simulink model "wireless_networked_control_HIL"  (Simulink 10.2)
settings: Solver=ode4  StartTime=0.0  StopTime=TfR  FixedStep=delta_t  RelTol=1e-3  EnableMultiTasking=on
values from neighbouring files (symbols this model uses):
  A1 = 0.01    [CoupledTanks_state_main.m]    (also in CoupledTanks_state_main_noise.m)
  A2 = 0.006    [CoupledTanks_state_main.m]    (also in CoupledTanks_state_main_noise.m)
  A3 = 0.12    [CoupledTanks_state_main.m]    (also in CoupledTanks_state_main_noise.m)
  A4 = 0.007    [CoupledTanks_state_main.m]    (also in CoupledTanks_state_main_noise.m)
  alpha1 = 10    [CoupledTanks_state_main.m]    (also in CoupledTanks_state_main_noise.m)
  AR = 1    [Controllersfun.m]    (also in Controllersfun2.m; CoupledTanks_state_main.m; CoupledTanks_state_main_noise.m)
  AR1 = 1    [CoupledTanks_state_main.m]    (also in CoupledTanks_state_main_noise.m)
  Atrace = [link5f(yh*trace_count+1:(yh+1)*trace_count+200),     link2f(yh*trace_count+1:(yh+1)*trace_count+200),     link3f(yh*trace_count+1:(yh+1)*trace_count+200),     link8f(yh*trace_count+1:(yh+1)*trace_count+200)]    [CoupledTanks_state_main.m]    (also in CoupledTanks_state_main_noise.m = Atrace_first_half; Mediasfun.m = Atrace_second_half)
  delta_t = 1/system_rate    (= 0.00104166666667)    [CoupledTanks_state_main.m]    (also in CoupledTanks_state_main_noise.m)
  delta_tc = abs(randn(N,1))    [ADPS_fig2_execution_timeanalyse.m]    (also in CoupledTanks_state_main.m = 0.0416666666667; CoupledTanks_state_main_noise.m = 0.0416666666667)
  delta_tc2 = 1/sensing_rate2    (= 0.0416666666667)    [CoupledTanks_state_main.m]    (also in CoupledTanks_state_main_noise.m)
  delta_tr = 8/960    (= 0.00833333333333)    [CoupledTanks_state_main.m]    (also in CoupledTanks_state_main_noise.m)
  g = 9.8    [Controllersfun.m]    (also in Controllersfun2.m; CoupledTanks_state_main.m; CoupledTanks_state_main_noise.m; EKFsfun.m)
  L1ini = 6    [CoupledTanks_state_main.m]    (also in CoupledTanks_state_main_noise.m)
  L1sp = 8.4375    [CoupledTanks_state_main.m]    (also in CoupledTanks_state_main_noise.m)
  L1sp2 = 6.75    [CoupledTanks_state_main.m]    (also in CoupledTanks_state_main_noise.m)
  L2ini = 7    [CoupledTanks_state_main.m]    (also in CoupledTanks_state_main_noise.m)
  L2sp = 15    [CoupledTanks_state_main.m]    (also in CoupledTanks_state_main_noise.m)
  L2sp2 = 12    [CoupledTanks_state_main.m]    (also in CoupledTanks_state_main_noise.m)
  LiniEKF = [9,10,12]    [CoupledTanks_state_main.m]    (also in CoupledTanks_state_main_noise.m)
  LiniEKF2 = [6,7,8]    [CoupledTanks_state_main.m]    (also in CoupledTanks_state_main_noise.m)
  Llb = [0,0,0]    [CoupledTanks_state_main.m]    (also in CoupledTanks_state_main_noise.m)
  LRini = 8    [CoupledTanks_state_main.m]    (also in CoupledTanks_state_main_noise.m)
  Lub = [50,50,50]    [CoupledTanks_state_main.m]    (also in CoupledTanks_state_main_noise.m)
  noise_change = 0    [CoupledTanks_state_main.m]    (also in CoupledTanks_state_main_noise.m = 1)
  p12 = 1    [CoupledTanks_state_main.m]    (also in CoupledTanks_state_main_noise.m)
  p22 = 1    [CoupledTanks_state_main.m]    (also in CoupledTanks_state_main_noise.m)
  p2tap = 1    [CoupledTanks_state_main.m]    (also in CoupledTanks_state_main_noise.m)
  R1 = 0.0006    [CoupledTanks_state_main.m]    (also in CoupledTanks_state_main_noise.m)
  R1tap = 0.001    [CoupledTanks_state_main.m]    (also in CoupledTanks_state_main_noise.m)
  R2 = 0.0008    [CoupledTanks_state_main.m]    (also in CoupledTanks_state_main_noise.m)
  R3 = 0.0006    [CoupledTanks_state_main.m]    (also in CoupledTanks_state_main_noise.m)
  R4 = 0.0008    [CoupledTanks_state_main.m]    (also in CoupledTanks_state_main_noise.m)
  rho = 1000    [Controllersfun.m]    (also in Controllersfun2.m; CoupledTanks_state_main.m; CoupledTanks_state_main_noise.m; EKFsfun.m)
  scheduling_algorithm = 2    [CoupledTanks_state_main.m]    (also in CoupledTanks_state_main_noise.m)
  TraceS = trace1(yh*(Tf*system_rate+1)+1:(yh+1)*(Tf*system_rate+1)+1)    [CoupledTanks_state_main.m]    (also in CoupledTanks_state_main_noise.m)
  trigger = 0.0008    [CoupledTanks_state_main.m]    (also in CoupledTanks_state_main_noise.m)
  trigger2 = 0.0008    [CoupledTanks_state_main.m]    (also in CoupledTanks_state_main_noise.m)
  uini = 20    [CoupledTanks_state_main.m]    (also in CoupledTanks_state_main_noise.m)
  uini2 = 20    [CoupledTanks_state_main.m]    (also in CoupledTanks_state_main_noise.m)
  usp = -47.92572    [CoupledTanks_state_main.m]    (also in CoupledTanks_state_main_noise.m)
  usp2 = -42.866    [CoupledTanks_state_main.m]    (also in CoupledTanks_state_main_noise.m)
settings Model: Creator=Rhine  LastModifiedBy=DELL
settings SolverCC: AutoInsertRateTranBlk=on
settings DataIOCC: LimitDataPoints=on  SignalLoggingSaveFormat=Dataset
settings OptimizationCC: ExpressionDepthLimit=2147483647
settings DebuggingCC: SolverPrmCheckMsg=warning  StateNameClashWarn=warning

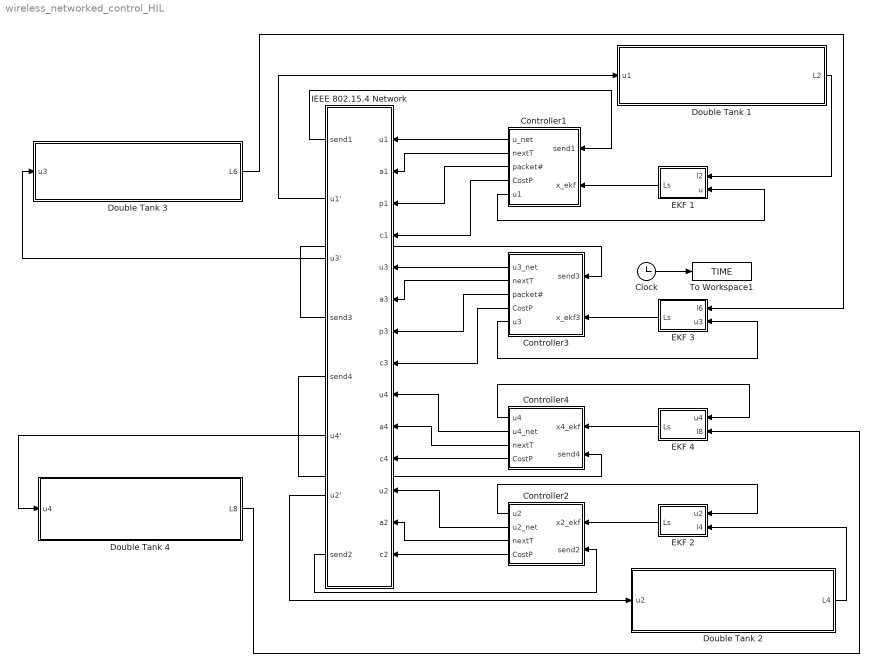
== system wireless_networked_control_HIL ==
  Clock : Clock
  Controller1 : Subsystem
  Controller2 : Subsystem
  Controller3 : Subsystem
  Controller4 : Subsystem
  Double Tank 1 : Subsystem
  Double Tank 2 : Subsystem
  Double Tank 3 : Subsystem
  "Double Tank 4 " : Subsystem
  EKF 1 : Subsystem
  EKF 2 : Subsystem
  EKF 3 : Subsystem
  EKF 4 : Subsystem
  IEEE 802.15.4 Network : Subsystem
  To Workspace1 : ToWorkspace  VariableName=TIME  SampleTime=-1
  wires:
  Clock/1 -> To Workspace1/1
  Controller1/1(u_net) -> IEEE 802.15.4 Network/1(u1)
  Controller1/2(nextT) -> IEEE 802.15.4 Network/2(a1)
  IEEE 802.15.4 Network/1(send1) -> Controller1/1(send1)
  Controller2/2(u2_net) -> IEEE 802.15.4 Network/12(u2)
  Controller2/3(nextT) -> IEEE 802.15.4 Network/13(a2)
  IEEE 802.15.4 Network/8(send2) -> Controller2/2(send2)
  Controller3/1(u3_net) -> IEEE 802.15.4 Network/5(u3)
  Controller3/2(nextT) -> IEEE 802.15.4 Network/6(a3)
  Controller4/2(u4_net) -> IEEE 802.15.4 Network/9(u4)
  Controller4/3(nextT) -> IEEE 802.15.4 Network/10(a4)
  IEEE 802.15.4 Network/4(send3) -> Controller3/1(send3)
  IEEE 802.15.4 Network/5(send4) -> Controller4/2(send4)
  Controller1/3(packet#) -> IEEE 802.15.4 Network/3(p1)
  Controller3/3(packet#) -> IEEE 802.15.4 Network/7(p3)
  Controller1/4(CostP) -> IEEE 802.15.4 Network/4(c1)
  Controller3/4(CostP) -> IEEE 802.15.4 Network/8(c3)
  Controller4/4(CostP) -> IEEE 802.15.4 Network/11(c4)
  Controller2/4(CostP) -> IEEE 802.15.4 Network/14(c2)
  IEEE 802.15.4 Network/3(u3') -> Double Tank 3/1(u3)
  IEEE 802.15.4 Network/2(u1') -> Double Tank 1/1(u1)
  IEEE 802.15.4 Network/6(u4') -> "Double Tank 4 "/1(u4)
  IEEE 802.15.4 Network/7(u2') -> Double Tank 2/1(u2)
  EKF 1/1(Ls) -> Controller1/2(x_ekf)
  Controller1/5(u1) -> EKF 1/2(u)
  Double Tank 1/1(L2) -> EKF 1/1(l2)
  EKF 3/1(Ls) -> Controller3/2(x_ekf3)
  Controller3/5(u3) -> EKF 3/2(u3)
  Double Tank 3/1(L6) -> EKF 3/1(l6)
  EKF 2/1(Ls) -> Controller2/1(x2_ekf)
  Double Tank 2/1(L4) -> EKF 2/2(l4)
  Controller2/1(u2) -> EKF 2/1(u2)
  EKF 4/1(Ls) -> Controller4/1(x4_ekf)
  Controller4/1(u4) -> EKF 4/1(u4)
  "Double Tank 4 "/1(L8) -> EKF 4/2(l8)

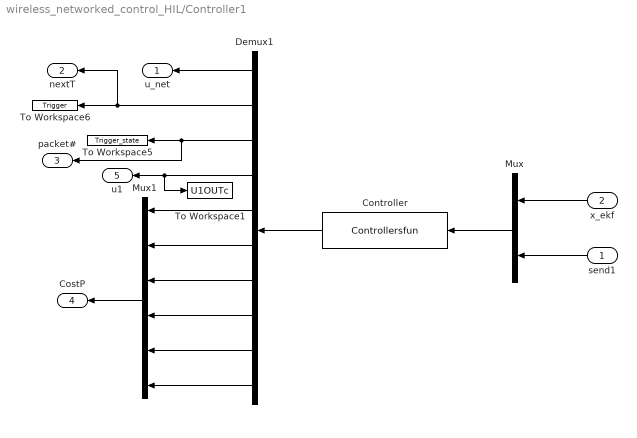
== system wireless_networked_control_HIL/Controller1 ==
  send1 : Inport
  x_ekf : Inport  Port=2
  Controller : S-Function  FunctionName=Controllersfun  Parameters=delta_t,delta_tc,A1,R1,A2,R2,alpha1,uini,trigger,L1sp,L2sp,usp  SFunctionDeploymentMode=off  EnableBusSupport=off
  Demux1 : Demux  Outputs=10
  Mux : Mux  Inputs=2
  Mux1 : Mux  Inputs=6
  To Workspace1 : ToWorkspace  VariableName=U1OUTc  SampleTime=-1
  To Workspace5 : ToWorkspace  VariableName=Trigger_state  SampleTime=-1
  To Workspace6 : ToWorkspace  VariableName=Trigger  SampleTime=-1
  u_net : Outport
  nextT : Outport  Port=2
  packet# : Outport  Port=3
  CostP : Outport  Port=4
  u1 : Outport  Port=5
  wires:
  Demux1/4 -> u1/1, To Workspace1/1
  Demux1/3 -> packet#/1, To Workspace5/1
  Controller/1 -> Demux1/1
  Demux1/2 -> nextT/1, To Workspace6/1
  Demux1/1 -> u_net/1
  x_ekf/1 -> Mux/1
  Mux/1 -> Controller/1
  send1/1 -> Mux/2
  Demux1/6 -> Mux1/2
  Demux1/5 -> Mux1/1
  Mux1/1 -> CostP/1
  Demux1/7 -> Mux1/3
  Demux1/8 -> Mux1/4
  Demux1/9 -> Mux1/5
  Demux1/10 -> Mux1/6

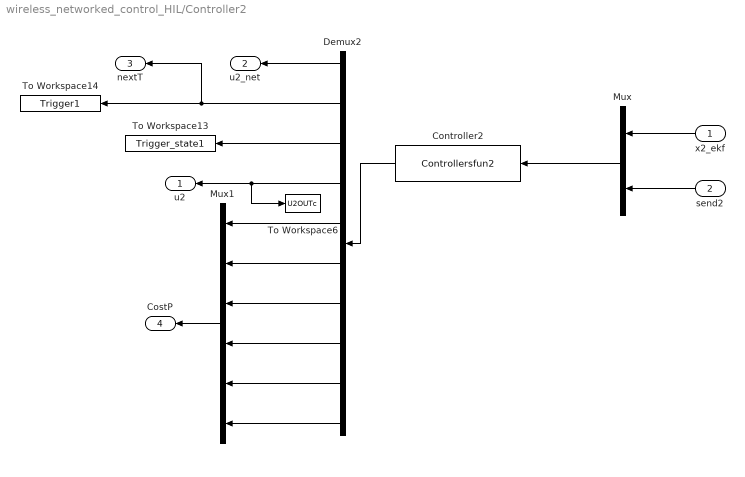
== system wireless_networked_control_HIL/Controller2 ==
  x2_ekf : Inport
  send2 : Inport  Port=2
  Controller2 : S-Function  FunctionName=Controllersfun2  Parameters=delta_t,delta_tc2,A3,R3,A4,R4,alpha1,uini2,trigger2,L1sp2,L2sp2,usp2  SFunctionDeploymentMode=off  EnableBusSupport=off
  Demux2 : Demux  Outputs=10
  Mux : Mux  Inputs=2
  Mux1 : Mux  Inputs=6
  To Workspace13 : ToWorkspace  VariableName=Trigger_state1  SampleTime=-1
  To Workspace14 : ToWorkspace  VariableName=Trigger1  SampleTime=-1
  To Workspace6 : ToWorkspace  VariableName=U2OUTc  SampleTime=-1
  u2 : Outport
  u2_net : Outport  Port=2
  nextT : Outport  Port=3
  CostP : Outport  Port=4
  wires:
  Demux2/4 -> u2/1, To Workspace6/1
  Demux2/3 -> To Workspace13/1
  Demux2/2 -> To Workspace14/1, nextT/1
  Demux2/1 -> u2_net/1
  Mux/1 -> Controller2/1
  Controller2/1 -> Demux2/1
  x2_ekf/1 -> Mux/1
  send2/1 -> Mux/2
  Mux1/1 -> CostP/1
  Demux2/5 -> Mux1/1
  Demux2/6 -> Mux1/2
  Demux2/7 -> Mux1/3
  Demux2/8 -> Mux1/4
  Demux2/9 -> Mux1/5
  Demux2/10 -> Mux1/6

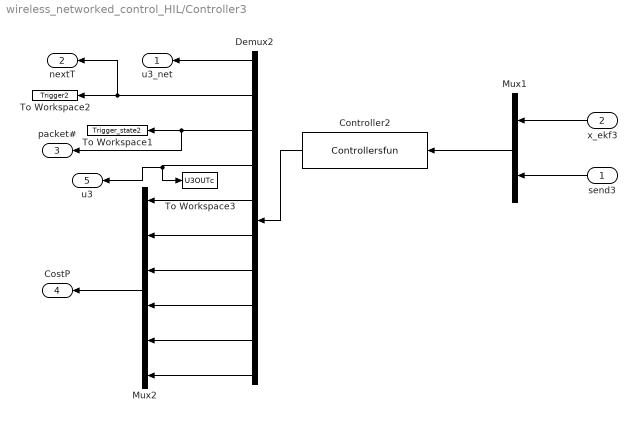
== system wireless_networked_control_HIL/Controller3 ==
  send3 : Inport
  x_ekf3 : Inport  Port=2
  Controller2 : S-Function  FunctionName=Controllersfun  Parameters=delta_t,delta_tc,A1,R1,A2,R2,alpha1,uini,trigger,L1sp,L2sp,usp  SFunctionDeploymentMode=off  EnableBusSupport=off
  Demux2 : Demux  Outputs=10
  Mux1 : Mux  Inputs=2
  Mux2 : Mux  Inputs=6
  To Workspace1 : ToWorkspace  VariableName=Trigger_state2  SampleTime=-1
  To Workspace2 : ToWorkspace  VariableName=Trigger2  SampleTime=-1
  To Workspace3 : ToWorkspace  VariableName=U3OUTc  SampleTime=-1
  u3_net : Outport
  nextT : Outport  Port=2
  packet# : Outport  Port=3
  CostP : Outport  Port=4
  u3 : Outport  Port=5
  wires:
  Mux2/1 -> CostP/1
  Demux2/2 -> nextT/1, To Workspace2/1
  Demux2/6 -> Mux2/2
  Controller2/1 -> Demux2/1
  Demux2/3 -> packet#/1, To Workspace1/1
  Demux2/1 -> u3_net/1
  Mux1/1 -> Controller2/1
  Demux2/4 -> u3/1, To Workspace3/1
  send3/1 -> Mux1/2
  x_ekf3/1 -> Mux1/1
  Demux2/5 -> Mux2/1
  Demux2/7 -> Mux2/3
  Demux2/8 -> Mux2/4
  Demux2/9 -> Mux2/5
  Demux2/10 -> Mux2/6

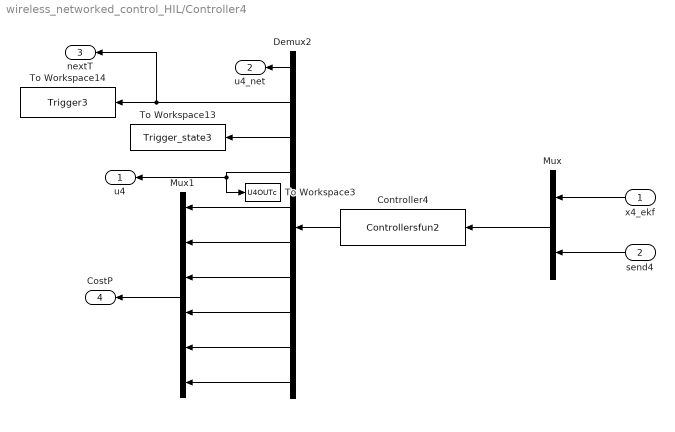
== system wireless_networked_control_HIL/Controller4 ==
  x4_ekf : Inport
  send4 : Inport  Port=2
  Controller4 : S-Function  FunctionName=Controllersfun2  Parameters=delta_t,delta_tc2,A3,R3,A4,R4,alpha1,uini2,trigger2,L1sp2,L2sp2,usp2  SFunctionDeploymentMode=off  EnableBusSupport=off
  Demux2 : Demux  Outputs=10
  Mux : Mux  Inputs=2
  Mux1 : Mux  Inputs=6
  To Workspace13 : ToWorkspace  VariableName=Trigger_state3  SampleTime=-1
  To Workspace14 : ToWorkspace  VariableName=Trigger3  SampleTime=-1
  To Workspace3 : ToWorkspace  VariableName=U4OUTc  SampleTime=-1
  u4 : Outport
  u4_net : Outport  Port=2
  nextT : Outport  Port=3
  CostP : Outport  Port=4
  wires:
  Demux2/4 -> u4/1, To Workspace3/1
  Demux2/3 -> To Workspace13/1
  Demux2/2 -> nextT/1, To Workspace14/1
  Demux2/1 -> u4_net/1
  Mux/1 -> Controller4/1
  Controller4/1 -> Demux2/1
  x4_ekf/1 -> Mux/1
  send4/1 -> Mux/2
  Mux1/1 -> CostP/1
  Demux2/5 -> Mux1/1
  Demux2/6 -> Mux1/2
  Demux2/7 -> Mux1/3
  Demux2/8 -> Mux1/4
  Demux2/9 -> Mux1/5
  Demux2/10 -> Mux1/6

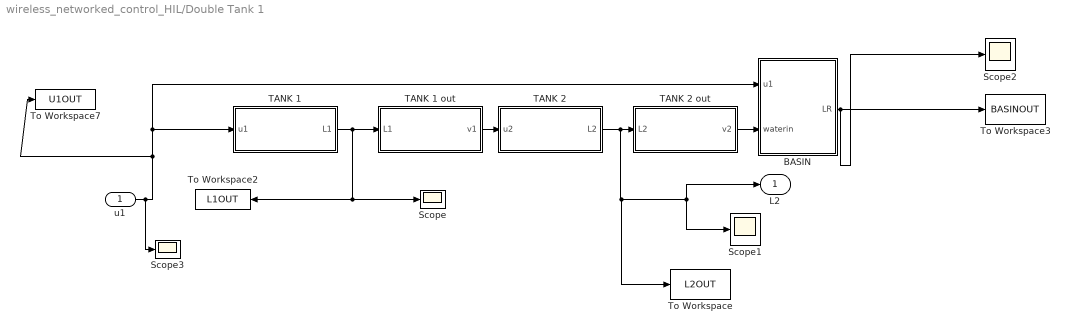
== system wireless_networked_control_HIL/Double Tank 1 ==
  u1 : Inport
  BASIN : Subsystem
  Scope{,1..3} (4 alike) : Scope
  TANK 1 : Subsystem
  TANK 1 out : Subsystem
  TANK 2 : Subsystem
  TANK 2 out : Subsystem
  To Workspace : ToWorkspace  VariableName=L2OUT  SampleTime=-1
  To Workspace2 : ToWorkspace  VariableName=L1OUT  SampleTime=-1
  To Workspace3 : ToWorkspace  VariableName=BASINOUT  SampleTime=-1
  To Workspace7 : ToWorkspace  VariableName=U1OUT  SampleTime=-1
  L2 : Outport
  wires:
  TANK 2 out/1(v2) -> BASIN/2(waterin)
  TANK 2/1(L2) -> To Workspace/1, L2/1, Scope1/1, TANK 2 out/1(L2)
  TANK 1 out/1(v1) -> TANK 2/1(u2)
  u1/1 -> Scope3/1, To Workspace7/1, BASIN/1(u1), TANK 1/1(u1)
  TANK 1/1(L1) -> Scope/1, To Workspace2/1, TANK 1 out/1(L1)
  BASIN/1(LR) -> Scope2/1, To Workspace3/1

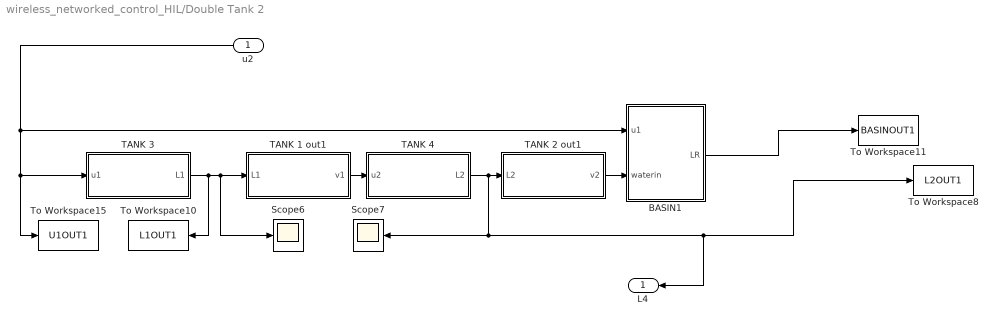
== system wireless_networked_control_HIL/Double Tank 2 ==
  u2 : Inport
  BASIN1 : Subsystem
  Scope6 : Scope
  Scope7 : Scope
  TANK 1 out1 : Subsystem
  TANK 2 out1 : Subsystem
  TANK 3 : Subsystem
  TANK 4 : Subsystem
  To Workspace10 : ToWorkspace  VariableName=L1OUT1  SampleTime=-1
  To Workspace11 : ToWorkspace  VariableName=BASINOUT1  SampleTime=-1
  To Workspace15 : ToWorkspace  VariableName=U1OUT1  SampleTime=-1
  To Workspace8 : ToWorkspace  VariableName=L2OUT1  SampleTime=-1
  L4 : Outport
  wires:
  TANK 3/1(L1) -> Scope6/1, TANK 1 out1/1(L1), To Workspace10/1
  TANK 1 out1/1(v1) -> TANK 4/1(u2)
  u2/1 -> To Workspace15/1, TANK 3/1(u1), BASIN1/1(u1)
  TANK 2 out1/1(v2) -> BASIN1/2(waterin)
  TANK 4/1(L2) -> TANK 2 out1/1(L2), L4/1, To Workspace8/1, Scope7/1
  BASIN1/1(LR) -> To Workspace11/1

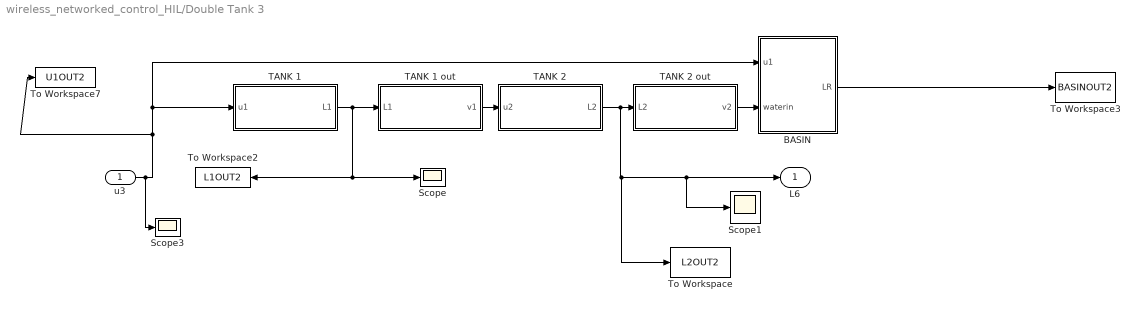
== system wireless_networked_control_HIL/Double Tank 3 ==
  u3 : Inport
  BASIN : Subsystem
  Scope : Scope
  Scope1 : Scope
  Scope3 : Scope
  TANK 1 : Subsystem
  TANK 1 out : Subsystem
  TANK 2 : Subsystem
  TANK 2 out : Subsystem
  To Workspace : ToWorkspace  VariableName=L2OUT2  SampleTime=-1
  To Workspace2 : ToWorkspace  VariableName=L1OUT2  SampleTime=-1
  To Workspace3 : ToWorkspace  VariableName=BASINOUT2  SampleTime=-1
  To Workspace7 : ToWorkspace  VariableName=U1OUT2  SampleTime=-1
  L6 : Outport
  wires:
  TANK 2 out/1(v2) -> BASIN/2(waterin)
  TANK 2/1(L2) -> To Workspace/1, L6/1, Scope1/1, TANK 2 out/1(L2)
  TANK 1 out/1(v1) -> TANK 2/1(u2)
  BASIN/1(LR) -> To Workspace3/1
  u3/1 -> Scope3/1, To Workspace7/1, BASIN/1(u1), TANK 1/1(u1)
  TANK 1/1(L1) -> Scope/1, To Workspace2/1, TANK 1 out/1(L1)

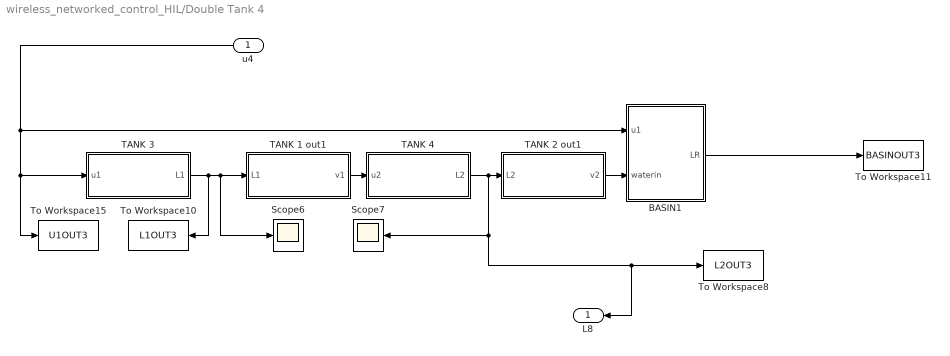
== system wireless_networked_control_HIL/Double Tank 4  ==
  u4 : Inport
  BASIN1 : Subsystem
  Scope6 : Scope
  Scope7 : Scope
  TANK 1 out1 : Subsystem
  TANK 2 out1 : Subsystem
  TANK 3 : Subsystem
  TANK 4 : Subsystem
  To Workspace10 : ToWorkspace  VariableName=L1OUT3  SampleTime=-1
  To Workspace11 : ToWorkspace  VariableName=BASINOUT3  SampleTime=-1
  To Workspace15 : ToWorkspace  VariableName=U1OUT3  SampleTime=-1
  To Workspace8 : ToWorkspace  VariableName=L2OUT3  SampleTime=-1
  L8 : Outport
  wires:
  TANK 3/1(L1) -> Scope6/1, TANK 1 out1/1(L1), To Workspace10/1
  TANK 1 out1/1(v1) -> TANK 4/1(u2)
  u4/1 -> To Workspace15/1, TANK 3/1(u1), BASIN1/1(u1)
  TANK 2 out1/1(v2) -> BASIN1/2(waterin)
  BASIN1/1(LR) -> To Workspace11/1
  TANK 4/1(L2) -> TANK 2 out1/1(L2), L8/1, To Workspace8/1, Scope7/1

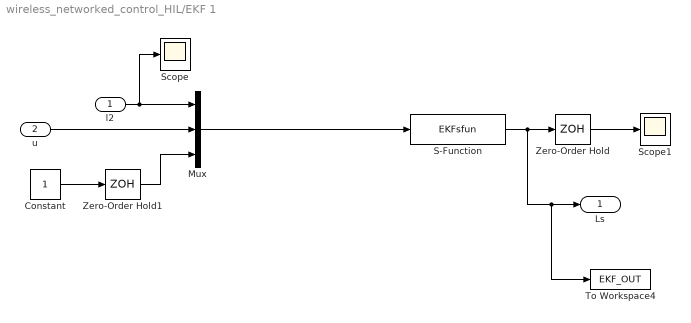
== system wireless_networked_control_HIL/EKF 1 ==
  l2 : Inport
  u : Inport  Port=2
  Constant : Constant
  Mux : Mux  Inputs=3
  S-Function : S-Function  FunctionName=EKFsfun  Parameters=delta_t,delta_tc,LiniEKF,TraceS,A1,R1,A2,R2,AR,alpha1  SFunctionDeploymentMode=off  EnableBusSupport=off
  Scope : Scope
  Scope1 : Scope
  To Workspace4 : ToWorkspace  VariableName=EKF_OUT  SampleTime=-1
  Zero-Order Hold : ZeroOrderHold  SampleTime=delta_t
  Zero-Order Hold1 : ZeroOrderHold  SampleTime=delta_t
  Ls : Outport
  wires:
  Mux/1 -> S-Function/1
  Zero-Order Hold1/1 -> Mux/3
  Constant/1 -> Zero-Order Hold1/1
  Zero-Order Hold/1 -> Scope1/1
  S-Function/1 -> Zero-Order Hold/1, Ls/1, To Workspace4/1
  u/1 -> Mux/2
  l2/1 -> Mux/1, Scope/1

== system wireless_networked_control_HIL/EKF 2 ==
  u2 : Inport
  l4 : Inport  Port=2
  Constant : Constant
  Mux : Mux  Inputs=3
  S-Function : S-Function  FunctionName=EKFsfun2  Parameters=delta_t,delta_tc2,LiniEKF2,TraceS,A3,R3,A4,R4,AR1,alpha1  SFunctionDeploymentMode=off  EnableBusSupport=off
  Scope : Scope
  Scope1 : Scope
  To Workspace12 : ToWorkspace  VariableName=EKF_OUT1  SampleTime=-1
  Zero-Order Hold : ZeroOrderHold  SampleTime=delta_t
  Zero-Order Hold1 : ZeroOrderHold  SampleTime=delta_t
  Ls : Outport
  wires:
  l4/1 -> Scope/1, Mux/1
  u2/1 -> Mux/2
  S-Function/1 -> To Workspace12/1, Ls/1, Zero-Order Hold/1
  Zero-Order Hold/1 -> Scope1/1
  Constant/1 -> Zero-Order Hold1/1
  Zero-Order Hold1/1 -> Mux/3
  Mux/1 -> S-Function/1

== system wireless_networked_control_HIL/EKF 3 ==
  l6 : Inport
  u3 : Inport  Port=2
  Constant : Constant
  Mux : Mux  Inputs=3
  S-Function : S-Function  FunctionName=EKFsfun3  Parameters=delta_t,delta_tc,LiniEKF,TraceS,A1,R1,A2,R2,AR,alpha1  SFunctionDeploymentMode=off  EnableBusSupport=off
  Scope : Scope
  Scope1 : Scope
  To Workspace4 : ToWorkspace  VariableName=EKF_OUT2  SampleTime=-1
  Zero-Order Hold : ZeroOrderHold  SampleTime=delta_t
  Zero-Order Hold1 : ZeroOrderHold  SampleTime=delta_t
  Ls : Outport
  wires:
  l6/1 -> Scope/1, Mux/1
  u3/1 -> Mux/2
  S-Function/1 -> To Workspace4/1, Ls/1, Zero-Order Hold/1
  Zero-Order Hold/1 -> Scope1/1
  Constant/1 -> Zero-Order Hold1/1
  Zero-Order Hold1/1 -> Mux/3
  Mux/1 -> S-Function/1

== system wireless_networked_control_HIL/EKF 4 ==
  u4 : Inport
  l8 : Inport  Port=2
  Constant : Constant
  Mux : Mux  Inputs=3
  S-Function : S-Function  FunctionName=EKFsfun4  Parameters=delta_t,delta_tc2,LiniEKF2,TraceS,A3,R3,A4,R4,AR1,alpha1  SFunctionDeploymentMode=off  EnableBusSupport=off
  Scope : Scope
  Scope1 : Scope
  To Workspace12 : ToWorkspace  VariableName=EKF_OUT3  SampleTime=-1
  Zero-Order Hold : ZeroOrderHold  SampleTime=delta_t
  Zero-Order Hold1 : ZeroOrderHold  SampleTime=delta_t
  Ls : Outport
  wires:
  l8/1 -> Scope/1, Mux/1
  u4/1 -> Mux/2
  S-Function/1 -> To Workspace12/1, Ls/1, Zero-Order Hold/1
  Zero-Order Hold/1 -> Scope1/1
  Constant/1 -> Zero-Order Hold1/1
  Zero-Order Hold1/1 -> Mux/3
  Mux/1 -> S-Function/1

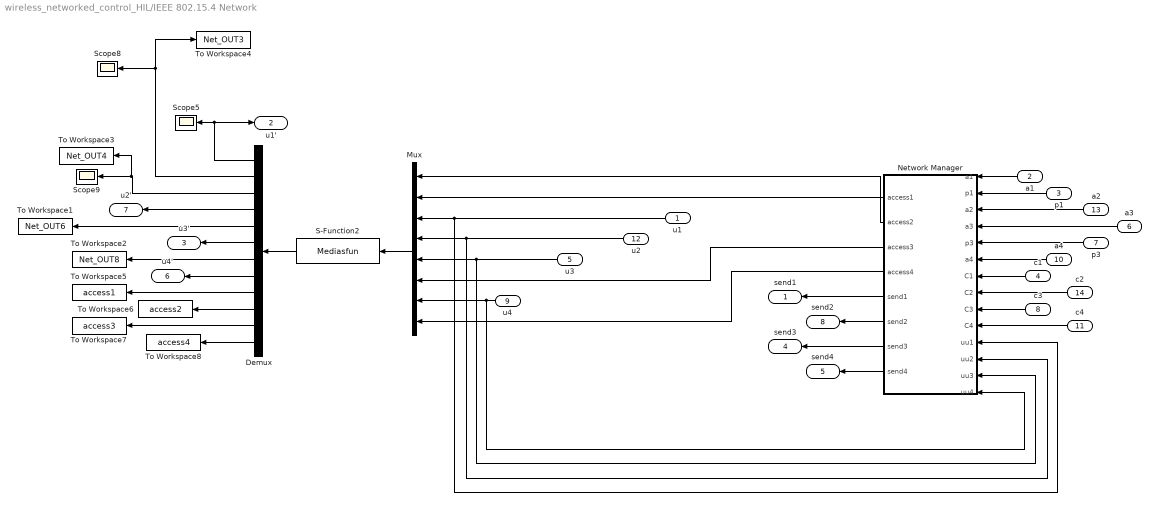
== system wireless_networked_control_HIL/IEEE 802.15.4 Network ==
  u1 : Inport
  a1 : Inport  Port=2
  p1 : Inport  Port=3
  c1 : Inport  Port=4
  u3 : Inport  Port=5
  a3 : Inport  Port=6
  p3 : Inport  Port=7
  c3 : Inport  Port=8
  u4 : Inport  Port=9
  a4 : Inport  Port=10
  c4 : Inport  Port=11
  u2 : Inport  Port=12
  a2 : Inport  Port=13
  c2 : Inport  Port=14
  Demux : Demux  Outputs=12
  Mux : Mux  Inputs=8
  Network Manager : Subsystem
  S-Function2 : S-Function  FunctionName=Mediasfun  Parameters=delta_t,delta_tr,delta_tc,delta_tc2,uini,Atrace,noise_change  SFunctionDeploymentMode=off  EnableBusSupport=off
  Scope5 : Scope
  Scope8 : Scope
  Scope9 : Scope
  To Workspace1 : ToWorkspace  VariableName=Net_OUT6  SampleTime=-1
  To Workspace2 : ToWorkspace  VariableName=Net_OUT8  SampleTime=-1
  To Workspace3 : ToWorkspace  VariableName=Net_OUT4  SampleTime=-1
  To Workspace4 : ToWorkspace  VariableName=Net_OUT3  SampleTime=-1
  To Workspace5 : ToWorkspace  VariableName=access1  SampleTime=-1
  To Workspace6 : ToWorkspace  VariableName=access2  SampleTime=-1
  To Workspace7 : ToWorkspace  VariableName=access3  SampleTime=-1
  To Workspace8 : ToWorkspace  VariableName=access4  SampleTime=-1
  send1 : Outport
  u1' : Outport  Port=2
  u3' : Outport  Port=3
  send3 : Outport  Port=4
  send4 : Outport  Port=5
  u4' : Outport  Port=6
  u2' : Outport  Port=7
  send2 : Outport  Port=8
  wires:
  u1/1 -> Network Manager/11(uu1), Mux/3
  u2/1 -> Network Manager/12(uu2), Mux/4
  Mux/1 -> S-Function2/1
  Network Manager/2(access2) -> Mux/2
  Network Manager/1(access1) -> Mux/1
  Network Manager/5(send1) -> send1/1
  Network Manager/6(send2) -> send2/1
  a1/1 -> Network Manager/1(a1)
  a2/1 -> Network Manager/3(a2)
  a3/1 -> Network Manager/4(a3)
  a4/1 -> Network Manager/6(a4)
  u3/1 -> Network Manager/13(uu3), Mux/5
  u4/1 -> Network Manager/14(uu4), Mux/7
  Network Manager/3(access3) -> Mux/6
  Network Manager/4(access4) -> Mux/8
  Network Manager/7(send3) -> send3/1
  Network Manager/8(send4) -> send4/1
  Demux/1 -> u1'/1, Scope5/1
  Demux/2 -> Scope8/1, To Workspace4/1
  Demux/12 -> To Workspace8/1
  Demux/6 -> u3'/1
  Demux/4 -> u2'/1
  Demux/5 -> To Workspace1/1
  Demux/8 -> u4'/1
  S-Function2/1 -> Demux/1
  Demux/3 -> To Workspace3/1, Scope9/1
  Demux/9 -> To Workspace5/1
  Demux/11 -> To Workspace7/1
  Demux/7 -> To Workspace2/1
  Demux/10 -> To Workspace6/1
  p1/1 -> Network Manager/2(p1)
  p3/1 -> Network Manager/5(p3)
  c1/1 -> Network Manager/7(C1)
  c2/1 -> Network Manager/8(C2)
  c3/1 -> Network Manager/9(C3)
  c4/1 -> Network Manager/10(C4)

== system wireless_networked_control_HIL/Double Tank 1/BASIN ==
  u1 : Inport
  waterin : Inport  Port=2
  Mux : Mux  Inputs=2
  S-Function : S-Function  FunctionName=BASINsfun  Parameters=alpha1,AR,Lub,Llb,rho,LRini  SFunctionDeploymentMode=off  EnableBusSupport=off
  Zero-Order Hold : ZeroOrderHold  SampleTime=delta_t
  LR : Outport
  wires:
  S-Function/1 -> Zero-Order Hold/1
  u1/1 -> Mux/1
  waterin/1 -> Mux/2
  Mux/1 -> S-Function/1
  Zero-Order Hold/1 -> LR/1

== system wireless_networked_control_HIL/Double Tank 1/TANK 1 ==
  u1 : Inport
  S-Function1 : S-Function  FunctionName=Tank1Sfun  Parameters=A1,Lub,rho,alpha1,R1,p12,R1tap,p2tap,g,L1ini  SFunctionDeploymentMode=off  EnableBusSupport=off
  Zero-Order Hold : ZeroOrderHold  SampleTime=delta_t
  L1 : Outport
  wires:
  S-Function1/1 -> Zero-Order Hold/1
  u1/1 -> S-Function1/1
  Zero-Order Hold/1 -> L1/1

== system wireless_networked_control_HIL/Double Tank 1/TANK 1 out ==
  L1 : Inport
  S-Function : S-Function  FunctionName=pipe1sfun  Parameters=rho,R1,p12,g  SFunctionDeploymentMode=off  EnableBusSupport=off
  v1 : Outport
  wires:
  L1/1 -> S-Function/1
  S-Function/1 -> v1/1

== system wireless_networked_control_HIL/Double Tank 1/TANK 2 ==
  u2 : Inport
  S-Function : S-Function  FunctionName=Tank2sfun  Parameters=A2,Lub,rho,R2,p22,g,L2ini  SFunctionDeploymentMode=off  EnableBusSupport=off
  Zero-Order Hold : ZeroOrderHold  SampleTime=delta_t
  L2 : Outport
  wires:
  u2/1 -> S-Function/1
  S-Function/1 -> Zero-Order Hold/1
  Zero-Order Hold/1 -> L2/1

== system wireless_networked_control_HIL/Double Tank 1/TANK 2 out ==
  L2 : Inport
  S-Function : S-Function  FunctionName=pipe2sfun  Parameters=rho,R2,p22,g  SFunctionDeploymentMode=off  EnableBusSupport=off
  v2 : Outport
  wires:
  L2/1 -> S-Function/1
  S-Function/1 -> v2/1

== system wireless_networked_control_HIL/Double Tank 2/BASIN1 ==
  u1 : Inport
  waterin : Inport  Port=2
  Mux : Mux  Inputs=2
  S-Function : S-Function  FunctionName=BASINsfun  Parameters=alpha1,AR1,Lub,Llb,rho,LRini  SFunctionDeploymentMode=off  EnableBusSupport=off
  Zero-Order Hold : ZeroOrderHold  SampleTime=delta_t
  LR : Outport
  wires:
  S-Function/1 -> Zero-Order Hold/1
  u1/1 -> Mux/1
  waterin/1 -> Mux/2
  Mux/1 -> S-Function/1
  Zero-Order Hold/1 -> LR/1

== system wireless_networked_control_HIL/Double Tank 2/TANK 1 out1 ==
  L1 : Inport
  S-Function : S-Function  FunctionName=pipe1sfun  Parameters=rho,R3,p12,g  SFunctionDeploymentMode=off  EnableBusSupport=off
  v1 : Outport
  wires:
  L1/1 -> S-Function/1
  S-Function/1 -> v1/1

== system wireless_networked_control_HIL/Double Tank 2/TANK 2 out1 ==
  L2 : Inport
  S-Function : S-Function  FunctionName=pipe2sfun  Parameters=rho,R4,p22,g  SFunctionDeploymentMode=off  EnableBusSupport=off
  v2 : Outport
  wires:
  L2/1 -> S-Function/1
  S-Function/1 -> v2/1

== system wireless_networked_control_HIL/Double Tank 2/TANK 3 ==
  u1 : Inport
  S-Function1 : S-Function  FunctionName=Tank1Sfun1  Parameters=A3,Lub,rho,alpha1,R3,p12,R1tap,p2tap,g,L1ini  SFunctionDeploymentMode=off  EnableBusSupport=off
  Zero-Order Hold : ZeroOrderHold  SampleTime=delta_t
  L1 : Outport
  wires:
  S-Function1/1 -> Zero-Order Hold/1
  u1/1 -> S-Function1/1
  Zero-Order Hold/1 -> L1/1

== system wireless_networked_control_HIL/Double Tank 2/TANK 4 ==
  u2 : Inport
  S-Function : S-Function  FunctionName=Tank2sfun1  Parameters=A4,Lub,rho,R4,p22,g,L2ini  SFunctionDeploymentMode=off  EnableBusSupport=off
  Zero-Order Hold : ZeroOrderHold  SampleTime=delta_t
  L2 : Outport
  wires:
  u2/1 -> S-Function/1
  S-Function/1 -> Zero-Order Hold/1
  Zero-Order Hold/1 -> L2/1

== system wireless_networked_control_HIL/Double Tank 3/BASIN ==
  u1 : Inport
  waterin : Inport  Port=2
  Mux : Mux  Inputs=2
  S-Function : S-Function  FunctionName=BASINsfun  Parameters=alpha1,AR,Lub,Llb,rho,LRini  SFunctionDeploymentMode=off  EnableBusSupport=off
  Zero-Order Hold : ZeroOrderHold  SampleTime=delta_t
  LR : Outport
  wires:
  S-Function/1 -> Zero-Order Hold/1
  u1/1 -> Mux/1
  waterin/1 -> Mux/2
  Mux/1 -> S-Function/1
  Zero-Order Hold/1 -> LR/1

== system wireless_networked_control_HIL/Double Tank 3/TANK 1 ==
  u1 : Inport
  S-Function1 : S-Function  FunctionName=Tank1Sfun  Parameters=A1,Lub,rho,alpha1,R1,p12,R1tap,p2tap,g,L1ini  SFunctionDeploymentMode=off  EnableBusSupport=off
  Zero-Order Hold : ZeroOrderHold  SampleTime=delta_t
  L1 : Outport
  wires:
  S-Function1/1 -> Zero-Order Hold/1
  u1/1 -> S-Function1/1
  Zero-Order Hold/1 -> L1/1

== system wireless_networked_control_HIL/Double Tank 3/TANK 1 out ==
  L1 : Inport
  S-Function : S-Function  FunctionName=pipe1sfun  Parameters=rho,R1,p12,g  SFunctionDeploymentMode=off  EnableBusSupport=off
  v1 : Outport
  wires:
  L1/1 -> S-Function/1
  S-Function/1 -> v1/1

== system wireless_networked_control_HIL/Double Tank 3/TANK 2 ==
  u2 : Inport
  S-Function : S-Function  FunctionName=Tank2sfun  Parameters=A2,Lub,rho,R2,p22,g,L2ini  SFunctionDeploymentMode=off  EnableBusSupport=off
  Zero-Order Hold : ZeroOrderHold  SampleTime=delta_t
  L2 : Outport
  wires:
  u2/1 -> S-Function/1
  S-Function/1 -> Zero-Order Hold/1
  Zero-Order Hold/1 -> L2/1

== system wireless_networked_control_HIL/Double Tank 3/TANK 2 out ==
  L2 : Inport
  S-Function : S-Function  FunctionName=pipe2sfun  Parameters=rho,R2,p22,g  SFunctionDeploymentMode=off  EnableBusSupport=off
  v2 : Outport
  wires:
  L2/1 -> S-Function/1
  S-Function/1 -> v2/1

== system wireless_networked_control_HIL/Double Tank 4 /BASIN1 ==
  u1 : Inport
  waterin : Inport  Port=2
  Mux : Mux  Inputs=2
  S-Function : S-Function  FunctionName=BASINsfun  Parameters=alpha1,AR1,Lub,Llb,rho,LRini  SFunctionDeploymentMode=off  EnableBusSupport=off
  Zero-Order Hold : ZeroOrderHold  SampleTime=delta_t
  LR : Outport
  wires:
  S-Function/1 -> Zero-Order Hold/1
  u1/1 -> Mux/1
  waterin/1 -> Mux/2
  Mux/1 -> S-Function/1
  Zero-Order Hold/1 -> LR/1

== system wireless_networked_control_HIL/Double Tank 4 /TANK 1 out1 ==
  L1 : Inport
  S-Function : S-Function  FunctionName=pipe1sfun  Parameters=rho,R3,p12,g  SFunctionDeploymentMode=off  EnableBusSupport=off
  v1 : Outport
  wires:
  L1/1 -> S-Function/1
  S-Function/1 -> v1/1

== system wireless_networked_control_HIL/Double Tank 4 /TANK 2 out1 ==
  L2 : Inport
  S-Function : S-Function  FunctionName=pipe2sfun  Parameters=rho,R4,p22,g  SFunctionDeploymentMode=off  EnableBusSupport=off
  v2 : Outport
  wires:
  L2/1 -> S-Function/1
  S-Function/1 -> v2/1

== system wireless_networked_control_HIL/Double Tank 4 /TANK 3 ==
  u1 : Inport
  S-Function1 : S-Function  FunctionName=Tank1Sfun1  Parameters=A3,Lub,rho,alpha1,R3,p12,R1tap,p2tap,g,L1ini  SFunctionDeploymentMode=off  EnableBusSupport=off
  Zero-Order Hold : ZeroOrderHold  SampleTime=delta_t
  L1 : Outport
  wires:
  S-Function1/1 -> Zero-Order Hold/1
  u1/1 -> S-Function1/1
  Zero-Order Hold/1 -> L1/1

== system wireless_networked_control_HIL/Double Tank 4 /TANK 4 ==
  u2 : Inport
  S-Function : S-Function  FunctionName=Tank2sfun1  Parameters=A4,Lub,rho,R4,p22,g,L2ini  SFunctionDeploymentMode=off  EnableBusSupport=off
  Zero-Order Hold : ZeroOrderHold  SampleTime=delta_t
  L2 : Outport
  wires:
  u2/1 -> S-Function/1
  S-Function/1 -> Zero-Order Hold/1
  Zero-Order Hold/1 -> L2/1

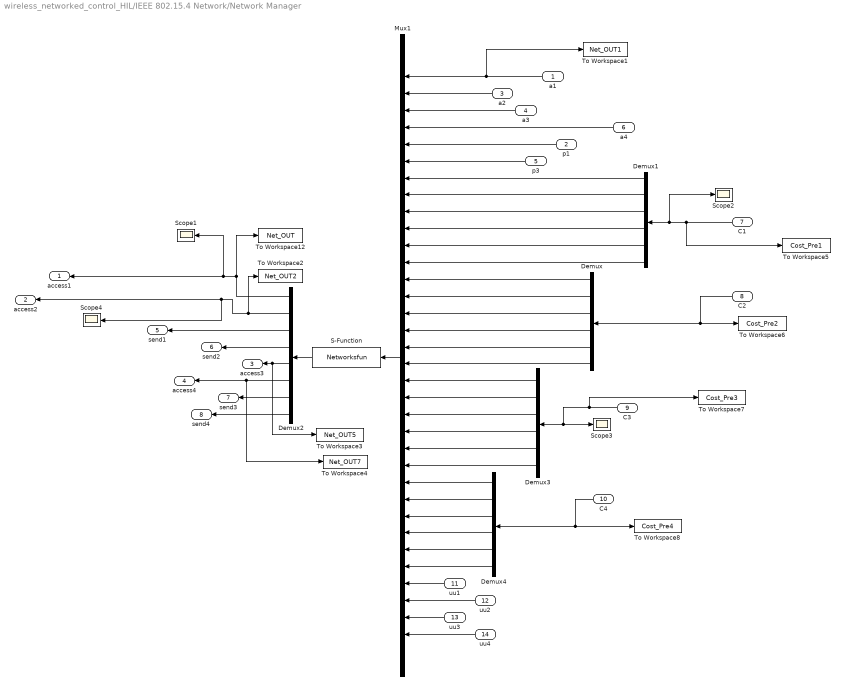
== system wireless_networked_control_HIL/IEEE 802.15.4 Network/Network Manager ==
  a1 : Inport
  p1 : Inport  Port=2
  a2 : Inport  Port=3
  a3 : Inport  Port=4
  p3 : Inport  Port=5
  a4 : Inport  Port=6
  C1 : Inport  Port=7
  C2 : Inport  Port=8
  C3 : Inport  Port=9
  C4 : Inport  Port=10
  uu1 : Inport  Port=11
  uu2 : Inport  Port=12
  uu3 : Inport  Port=13
  uu4 : Inport  Port=14
  Demux{,1,3..4} (4 alike) : Demux  Outputs=6
  Demux2 : Demux  Outputs=8
  Mux1 : Mux  Inputs=34
  S-Function : S-Function  FunctionName=Networksfun  Parameters=delta_t,delta_tr,delta_tc,delta_tc2,scheduling_algorithm  SFunctionDeploymentMode=off  EnableBusSupport=off
  Scope{1..4} (4 alike) : Scope
  To Workspace1 : ToWorkspace  VariableName=Net_OUT1  SampleTime=-1
  To Workspace12 : ToWorkspace  VariableName=Net_OUT  SampleTime=-1
  To Workspace2 : ToWorkspace  VariableName=Net_OUT2  SampleTime=-1
  To Workspace3 : ToWorkspace  VariableName=Net_OUT5  SampleTime=-1
  To Workspace4 : ToWorkspace  VariableName=Net_OUT7  SampleTime=-1
  To Workspace5 : ToWorkspace  VariableName=Cost_Pre1  SampleTime=-1
  To Workspace6 : ToWorkspace  VariableName=Cost_Pre2  SampleTime=-1
  To Workspace7 : ToWorkspace  VariableName=Cost_Pre3  SampleTime=-1
  To Workspace8 : ToWorkspace  VariableName=Cost_Pre4  SampleTime=-1
  access1 : Outport
  access2 : Outport  Port=2
  access3 : Outport  Port=3
  access4 : Outport  Port=4
  send1 : Outport  Port=5
  send2 : Outport  Port=6
  send3 : Outport  Port=7
  send4 : Outport  Port=8
  wires:
  S-Function/1 -> Demux2/1
  Mux1/1 -> S-Function/1
  Demux2/2 -> Scope4/1, access2/1, To Workspace2/1
  a1/1 -> To Workspace1/1, Mux1/1
  Demux2/1 -> To Workspace12/1, access1/1, Scope1/1
  Demux2/3 -> send1/1
  Demux2/4 -> send2/1
  Demux2/5 -> To Workspace3/1, access3/1
  Demux2/6 -> To Workspace4/1, access4/1
  Demux2/7 -> send3/1
  Demux2/8 -> send4/1
  a2/1 -> Mux1/2
  a3/1 -> Mux1/3
  a4/1 -> Mux1/4
  p1/1 -> Mux1/5
  p3/1 -> Mux1/6
  C1/1 -> Demux1/1, Scope2/1, To Workspace5/1
  Demux1/1 -> Mux1/7
  Demux1/2 -> Mux1/8
  C3/1 -> To Workspace7/1, Scope3/1, Demux3/1
  C4/1 -> To Workspace8/1, Demux4/1
  C2/1 -> Demux/1, To Workspace6/1
  Demux1/3 -> Mux1/9
  Demux1/4 -> Mux1/10
  Demux1/5 -> Mux1/11
  Demux1/6 -> Mux1/12
  Demux/1 -> Mux1/13
  Demux/2 -> Mux1/14
  Demux/3 -> Mux1/15
  Demux/4 -> Mux1/16
  Demux/5 -> Mux1/17
  Demux/6 -> Mux1/18
  Demux3/1 -> Mux1/19
  Demux3/2 -> Mux1/20
  Demux3/3 -> Mux1/21
  Demux3/4 -> Mux1/22
  Demux3/5 -> Mux1/23
  Demux3/6 -> Mux1/24
  Demux4/1 -> Mux1/25
  Demux4/2 -> Mux1/26
  Demux4/3 -> Mux1/27
  Demux4/4 -> Mux1/28
  Demux4/5 -> Mux1/29
  Demux4/6 -> Mux1/30
  uu1/1 -> Mux1/31
  uu2/1 -> Mux1/32
  uu3/1 -> Mux1/33
  uu4/1 -> Mux1/34
